simulink model "satellite_adcs_model"  (R2014b)
settings: Solver=ode3  SolverMode=SingleTasking  StartTime=0.0  StopTime=tdur  FixedStep=dt  RelTol=1e-3
undefined symbols (not defined in the file or in its folder): CTRL_DT_MODE, CTRL_PT_MODE, CTRL_SWITCH, dt, dt_gyro, dt_mg, dt_ss, dt_st, dt_ts, FOV, GYRO_Bias, magnitude, q_B_I_0, R_0, R_G_B, R_S1_B, R_S2_B, R_S3_B, R_S4_B, sigMag, sigSS, Taero_toggle, temp_coeff, temp_ref, Tgg_toggle, Tsolar_toggle, Ug, Umg, V_0, Var_ARW, Var_RRW, varST_x, varST_y, varST_z, varTemp, VarW, w_B_BI_0
libraries: simulink x6
(part 2 of 2)

== system satellite_adcs_model/Sensors/Sun Sensor/Sun Sensor 3 ==
  S_B_hat : Inport
  Compare To Constant1 : simulink/Logic and Bit Operations/Compare To Constant  relop=<=  const=-cos(FOV)  OutDataTypeStr=boolean
  Demux2 : Demux  Outputs=3
  Mux1 : Mux  Inputs=3
  Product : Product
  R_S3_B : Gain  Gain=R_S3_B  Multiplication=Matrix(K*u)
  SS Noise : RandomNumber  Variance=(sigSS*pi/180)^2  SampleTime=dt_ss
  Sum : Sum  Inputs=++|
  S_S3_m : Outport
  S_S3 : Outport  Port=2
  wires:
  Product/1 -> S_S3_m/1
  R_S3_B/1 -> S_S3/1, Demux2/1
  Demux2/1 -> Mux1/1
  Demux2/2 -> Mux1/2
  Demux2/3 -> Compare To Constant1/1, Mux1/3
  Compare To Constant1/1 -> Product/2
  S_B_hat/1 -> R_S3_B/1
  Sum/1 -> Product/1
  SS Noise/1 -> Sum/1
  Mux1/1 -> Sum/2

== system satellite_adcs_model/Sensors/Sun Sensor/Sun Sensor 4 ==
  S_B_hat : Inport
  Compare To Constant1 : simulink/Logic and Bit Operations/Compare To Constant  relop=<=  const=-cos(FOV)  OutDataTypeStr=boolean
  Demux2 : Demux  Outputs=3
  Mux1 : Mux  Inputs=3
  Product : Product
  R_S4_B*(u) : Gain  Gain=R_S4_B  Multiplication=Matrix(K*u)
  SS Noise : RandomNumber  Variance=(sigSS*pi/180)^2  SampleTime=dt_ss
  Sum : Sum  Inputs=++|
  S_S4_m : Outport
  S_S4 : Outport  Port=2
  wires:
  Product/1 -> S_S4_m/1
  R_S4_B*(u)/1 -> S_S4/1, Demux2/1
  Demux2/1 -> Mux1/1
  Demux2/2 -> Mux1/2
  Demux2/3 -> Compare To Constant1/1, Mux1/3
  Compare To Constant1/1 -> Product/2
  S_B_hat/1 -> R_S4_B*(u)/1
  Sum/1 -> Product/1
  SS Noise/1 -> Sum/1
  Mux1/1 -> Sum/2
